simulink model "PD_Notch_Final"  (R2018b)
settings: Solver=VariableStepAuto  StartTime=0.0  StopTime=100  RelTol=1e-3
libraries: slctrlblks x1, dspsrcs4 x1, simulink x1, cstblocks x1
settings Model: Creator=shrav  LastModifiedBy=shrav

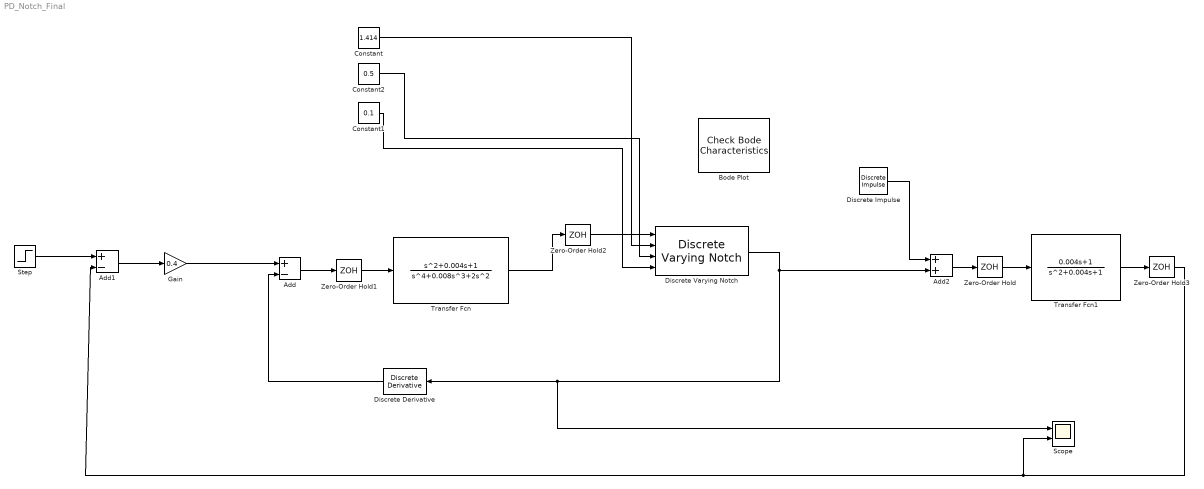
== system PD_Notch_Final ==
  Add : Sum  Inputs=+-
  Add1 : Sum  Inputs=+-
  Add2 : Sum
  Bode Plot : slctrlblks/Model Verification/Check Bode  Characteristics  InstantiateOnLoad=on  SaveOperatingPoints=off  LinearizationIOs={'/Step', 1, 'in', 'off', '';'/Zero-Order Hold2', 1, 'out', 'off', ''}  LinearizeAt=SnapshotTimes  SnapshotTimes=[0]  TriggerType=rising  SampleTime=auto  RateConversionMethod=zoh  PreWarpFreq=10  UseExactDelayModel=off  UseFullBlockNameLabels=off  UseBusSignalLabels=off  enabled=on  stopWhenAssertionFail=off  export=off  ViewDlgPos=[359 159 1062 638]  OpenViewOnLoad=off  LaunchViewOnOpen=off  FrequencyUnits=rad/s  MagnitudeUnits=dB  PhaseUnits=deg  TimeUnits=seconds  EnableUpperBound=off  UpperBoundFrequencies=[]  UpperBoundMagnitudes=[]  EnableLowerBound=off  LowerBoundFrequencies=[]  LowerBoundMagnitudes=[]
      settings: SourceProductName=Simulink Control Design
  Constant : Constant  Value=1.414
  Constant1 : Constant  Value=0.1
  Constant2 : Constant  Value=0.5
  Discrete Impulse : dspsrcs4/Discrete  Impulse  Delay=0  SampleTime=0.001  FrameSample=1  OutputFrames=off  dataType=double  isSigned=on  wordLen=16  udDataType=sfix(16)  fracBitsMode=Best precision  numFracBits=15  OutDataTypeStr=double  LastOutDataTypeStr=double
  Discrete Derivative : simulink/Discrete/Discrete Derivative  gainval=1  ICPrevScaledInput=0.0  OutMin=[]  OutMax=[]  OutDataType=fixdt(1, 16)  OutScaling=2^-10  DoSatur=off
  Discrete Varying Notch : cstblocks/Linear Parameter Varying/Discrete Varying Notch  w0=0  Ts=0.01
      settings: SourceProductName=Control System Toolbox  SourceProductBaseCode=CT
  Gain : Gain  Gain=0.4
  Scope : Scope  NumInputPorts=2
  Step : Step  Time=0  SampleTime=0.01
  Transfer Fcn : TransferFcn  Numerator=[1 0.004 1]  Denominator=[1 0.008 2 0 0]
  Transfer Fcn1 : TransferFcn  Numerator=[0.004 1]  Denominator=[1 0.004 1]
  Zero-Order Hold{,1..3} (4 alike) : ZeroOrderHold  SampleTime=-1
  wires:
  Discrete Derivative/1 -> Add/2
  Step/1 -> Add1/1
  Add/1 -> Zero-Order Hold1/1
  Zero-Order Hold1/1 -> Transfer Fcn/1
  Zero-Order Hold/1 -> Transfer Fcn1/1
  Add2/1 -> Zero-Order Hold/1
  Discrete Varying Notch/1 -> Discrete Derivative/1, Scope/1, Add2/2
  Transfer Fcn1/1 -> Zero-Order Hold3/1
  Constant2/1 -> Discrete Varying Notch/3
  Constant/1 -> Discrete Varying Notch/2
  Constant1/1 -> Discrete Varying Notch/4
  Add1/1 -> Gain/1
  Transfer Fcn/1 -> Zero-Order Hold2/1
  Zero-Order Hold2/1 -> Discrete Varying Notch/1
  Discrete Impulse/1 -> Add2/1
  Gain/1 -> Add/1
  Zero-Order Hold3/1 -> Scope/2, Add1/2
